simulink model "untitled1"  (Simulink 7.9)
settings: Solver=ode45  StartTime=0.0  StopTime=1  RelTol=1e-3
values from neighbouring files (symbols this model uses):
  D = [  1 -1  1 -1  1  1 -1 -1 ... (first row only)    [cdma.m]    (also in compressed_sampling.m = idct(eye(5000,5000)))
  j = imread('lena.jpg')    [ansk3.m]    (also in cosine_filter.m = 2; imag1.m)
undefined symbols (not defined in the file or in its folder): dfilt, F_nco, OFDM_Frame, Pilot_Level, QAM_Level
libraries: dspobslib x4, dspsigops x4, simulink x2, dsparch4 x1, commrandsrc2 x1, dspxfrm3 x1, commdigbbndam3 x1, dspstat3 x1
settings Model: Creator=ArunKB

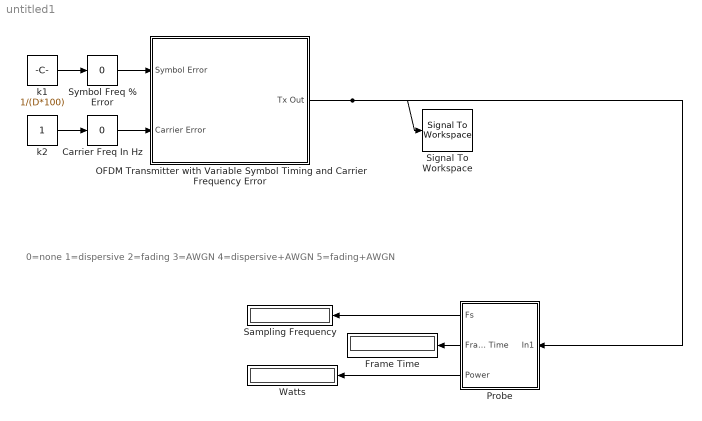
== system untitled1 ==
  note: 0=none
      | 1=dispersive
      | 2=fading
      | 3=AWGN
      | 4=dispersive+AWGN
      | 5=fading+AWGN
  Carrier Freq In Hz : simulink/Math Operations/Slider Gain  low=-1000  gain=0  high=1000
  Frame Time : Display
  OFDM Transmitter with Variable Symbol Timing and Carrier Frequency Error : Subsystem
  Probe : Subsystem
  Sampling Frequency : Display
  Signal To Workspace : SignalToWorkspace  VariableName=yout
      settings: CopyFcn=dspblkcopystw(gcbh);
  "Symbol Freq % Error " : simulink/Math Operations/Slider Gain  low=-0.5  gain=0  high=0.5
  Watts : Display
  k1 : Constant  Value=1/(D*100)
  k2 : Constant
  wires:
  k1/1 -> "Symbol Freq % Error "/1
  "Symbol Freq % Error "/1 -> OFDM Transmitter with Variable Symbol Timing and Carrier Frequency Error/1(Symbol Error)
  k2/1 -> Carrier Freq In Hz/1
  Carrier Freq In Hz/1 -> OFDM Transmitter with Variable Symbol Timing and Carrier Frequency Error/2(Carrier Error)
  OFDM Transmitter with Variable Symbol Timing and Carrier Frequency Error/1(Tx Out) -> Signal To Workspace/1, Probe/1(In1)
  Probe/1(Fs) -> Sampling Frequency/1
  Probe/3(Power) -> Watts/1
  Probe/2(Frame Time) -> Frame Time/1

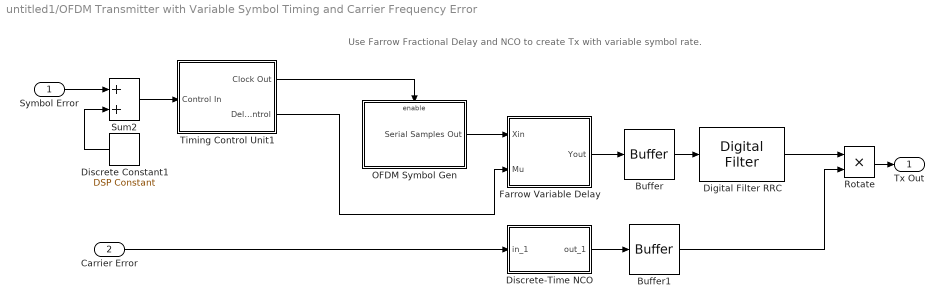
== system untitled1/OFDM Transmitter with Variable Symbol Timing and Carrier Frequency Error ==
  note: Use Farrow Fractional Delay and NCO to create Tx with variable symbol rate.
  Symbol Error : Inport
  Carrier Error : Inport  Port=2
  Buffer : Buffer  N=OFDM_Frame*D
  Buffer1 : Buffer  N=OFDM_Frame*D
  "Digital Filter RRC " : dsparch4/Digital Filter  TypePopup=FIR (all zeros)  IIRFiltStruct=Direct form II transposed  AllPoleFiltStruct=Direct form  FIRFiltStruct=Direct form  CoeffSource=Specify via dialog  NumCoeffs=rrc_coef  DenCoeffs=[1 0.1]  BiQuadCoeffs=[1 0.3 0.4 1 0.1 0.2]  LatticeCoeffs=[0.2 0.4]  denIgnore=on  FiltPerSampPopup=One filter per frame  IC=0  ICnum=0  ICden=0  roundingMode=Floor  overflowMode=off  ScaleValues=1  scaleValueFracLength=14  stageInFracLength=15  stageOutFracLength=15  FilterSource=Specify via dialog  dfiltObjectName=dfilt.dffir([1 2 1])  InputProcessing=Inherited (this choice will be removed - see release notes)
  Discrete Constant1 : dspobslib/DSP Constant  Value=1/D  SampleMode=Discrete  discreteOutput=Sample-based (interpret vectors as 1-D)  continuousOutput=Sample-based  sampTime=inf  framePeriod=inf  dataType=Inherit via back propagation  isSigned=on  wordLen=16  udDataType=sfix(16)  fracBitsMode=Best precision  numFracBits=15  InterpretAs1D=on  Ts=inf  FramebasedOutput=off
      settings: additionalParams=on
  Discrete-Time NCO : Subsystem  mask(Discrete-Time VCO){Ac=1, Fc=0, Kc=1, Ph=0, ts=1/F_nco}
      mask prompts: Ac "Output amplitude:"; Fc "Oscillation frequency (Hz):"; Kc "Input sensitivity:"; Ph "Initial phase (rad):"; ts "Sample time:"
      mask help: Generate a discrete-time output signal whose frequency changes in response to the amplitude variations of the input signal. The input signal must be a scalar.
      mask init:
      | if ((length(Ac)~=1) | (length(Fc)~=1) | (length(Kc)~=1) | (length(Ph)~=1) | (length(ts)~=1) |(length(Ph)~=1))error('Mask parameters must be scalar values.');end;
      | pi2=2*pi;
      mask Help: helpview(commbhelp)
      mask Display: disp('Discrete-Time\nNCO (rab)')
  Farrow Variable Delay : Subsystem
  OFDM Symbol Gen : Subsystem
  Rotate : Product  RndMeth=Zero
  Sum2 : Sum  SaturateOnIntegerOverflow=on  InputSameDT=on  OutDataTypeStr=Inherit: Same as first input
  Timing Control Unit1 : Subsystem
  Tx Out : Outport
  wires:
  Rotate/1 -> Tx Out/1
  Symbol Error/1 -> Sum2/1
  Farrow Variable Delay/1(Yout) -> Buffer/1
  Buffer/1 -> "Digital Filter RRC "/1
  "Digital Filter RRC "/1 -> Rotate/1
  Discrete-Time NCO/1(out_1) -> Buffer1/1
  Carrier Error/1 -> Discrete-Time NCO/1(in_1)
  Buffer1/1 -> Rotate/2
  Sum2/1 -> Timing Control Unit1/1(Control In)
  Timing Control Unit1/2(Delay Control) -> Farrow Variable Delay/2(Mu)
  Timing Control Unit1/1(Clock Out) -> OFDM Symbol Gen/Enable
  Discrete Constant1/1 -> Sum2/2
  OFDM Symbol Gen/1(Serial Samples Out) -> Farrow Variable Delay/1(Xin)

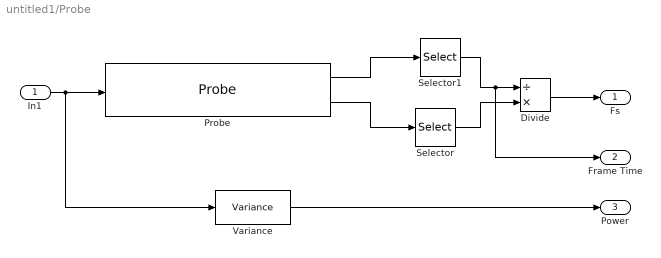
== system untitled1/Probe ==
  In1 : Inport
  Divide : Product  Inputs=/*
  Probe : Probe  ProbeWidth=off  ProbeComplexSignal=off  ProbeSignalDimensions=on
  Selector : Selector  InputPortWidth=2  IndexOptions=Index vector (dialog)  Indices=[1]  OutputSizes=1
  Selector1 : Selector  InputPortWidth=2  IndexOptions=Index vector (dialog)  Indices=[1]  OutputSizes=1
  Variance : dspstat3/Variance  run=off  reset_popup=None  InputProcessing=Columns as channels (frame based)  directionMode=Each column  dimension=1  treatSBRowAsCol=on  roiEnable=off  roiType=Rectangles  roiPortion=Entire ROI  roiOutput=Individual statistics for each ROI  roiFlag=off  roundingMode=Floor  overflowMode=off
  Fs : Outport
  Frame Time : Outport  Port=2
  Power : Outport  Port=3
  wires:
  In1/1 -> Probe/1, Variance/1
  Divide/1 -> Fs/1
  Selector/1 -> Divide/2
  Selector1/1 -> Divide/1, Frame Time/1
  Probe/1 -> Selector1/1
  Probe/2 -> Selector/1
  Variance/1 -> Power/1

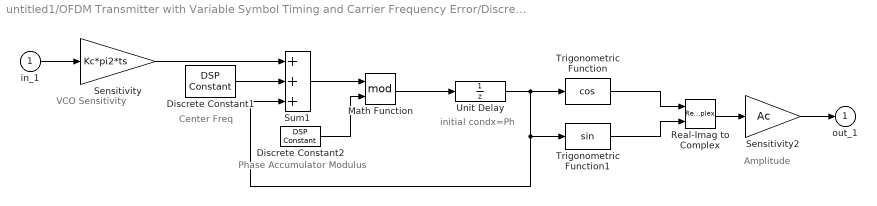
== system untitled1/OFDM Transmitter with Variable Symbol Timing and Carrier Frequency Error/Discrete-Time NCO ==
  note: initial condx=Ph
  note: VCO Sensitivity
  note: Center Freq
  note: Phase Accumulator
      | Modulus
  note: Amplitude
  in_1 : Inport
  Discrete Constant1 : dspobslib/DSP Constant  Value=Fc*pi2*ts  SampleMode=Discrete  discreteOutput=Sample-based (interpret vectors as 1-D)  continuousOutput=Sample-based  sampTime=ts  framePeriod=ts  dataType=Inherit via back propagation  isSigned=on  wordLen=16  udDataType=sfix(16)  fracBitsMode=Best precision  numFracBits=15  InterpretAs1D=on  Ts=ts  FramebasedOutput=off
      settings: additionalParams=on
  Discrete Constant2 : dspobslib/DSP Constant  Value=pi2  SampleMode=Discrete  discreteOutput=Sample-based (interpret vectors as 1-D)  continuousOutput=Sample-based  sampTime=ts  framePeriod=ts  dataType=Inherit via back propagation  isSigned=on  wordLen=16  udDataType=sfix(16)  fracBitsMode=Best precision  numFracBits=15  InterpretAs1D=on  Ts=ts  FramebasedOutput=off
      settings: additionalParams=on
  Math Function : Math  Operator=mod  SaturateOnIntegerOverflow=on
  Real-Imag to Complex : RealImagToComplex
  Sensitivity : Gain  Gain=Kc*pi2*ts  SaturateOnIntegerOverflow=on  OutDataTypeStr=Inherit: Same as input  ParamDataTypeStr=Inherit: Same as input
  Sensitivity2 : Gain  Gain=Ac  SaturateOnIntegerOverflow=on  OutDataTypeStr=Inherit: Same as input  ParamDataTypeStr=Inherit: Same as input
  Sum1 : Sum  Inputs=+++  SaturateOnIntegerOverflow=on  InputSameDT=on  OutDataTypeStr=Inherit: Same as first input
  Trigonometric Function : Trigonometry  Operator=cos
  Trigonometric Function1 : Trigonometry
  Unit Delay : UnitDelay  X0=Ph  SampleTime=ts
  out_1 : Outport  InitialOutput=0
  wires:
  Real-Imag to Complex/1 -> Sensitivity2/1
  Trigonometric Function1/1 -> Real-Imag to Complex/2
  Discrete Constant2/1 -> Math Function/2
  Sum1/1 -> Math Function/1
  Math Function/1 -> Unit Delay/1
  in_1/1 -> Sensitivity/1
  Sensitivity/1 -> Sum1/1
  Unit Delay/1 -> Trigonometric Function/1, Trigonometric Function1/1, Sum1/3
  Trigonometric Function/1 -> Real-Imag to Complex/1
  Sensitivity2/1 -> out_1/1
  Discrete Constant1/1 -> Sum1/2

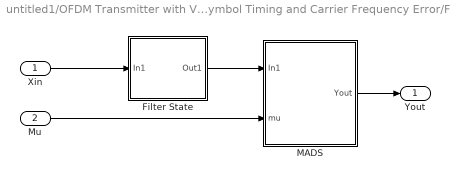
== system untitled1/OFDM Transmitter with Variable Symbol Timing and Carrier Frequency Error/Farrow Variable Delay ==
  Xin : Inport
  Mu : Inport  Port=2
  Filter State : Subsystem
  MADS : Subsystem
  Yout : Outport
  wires:
  Filter State/1(Out1) -> MADS/1(In1)
  Xin/1 -> Filter State/1(In1)
  Mu/1 -> MADS/2(mu)
  MADS/1(Yout) -> Yout/1

== system untitled1/OFDM Transmitter with Variable Symbol Timing and Carrier Frequency Error/OFDM Symbol Gen ==
  note: Output Samples Serially
  note: Note: Ouptut is SET TO ZERO
      | when not enabled.
      | This effecitvly inserts ZEROS in the stream
      | for proper interpolation.
  Enable : EnablePort
  Divide by  OFDM_Frame length : Subsystem  TreatAsAtomicUnit=on  mask(Pulse Divider){div=OFDM_Frame, ph=0}
      mask prompts: div "Modulo:"; ph "Initial Phase Delay (cycles):"
  OFDM Generator : Subsystem
  Selector : Selector  InputPortWidth=80  IndexOptions=Index vector (port)  Indices=[1 3]  OutputSizes=1
  Serial Samples Out : Outport  OutputWhenDisabled=reset  InitialOutput=0+j*eps
  wires:
  OFDM Generator/1(Out1) -> Selector/1
  Divide by  OFDM_Frame length/1(Enable) -> OFDM Generator/Enable
  Selector/1 -> Serial Samples Out/1
  Divide by  OFDM_Frame length/2(Count) -> Selector/2

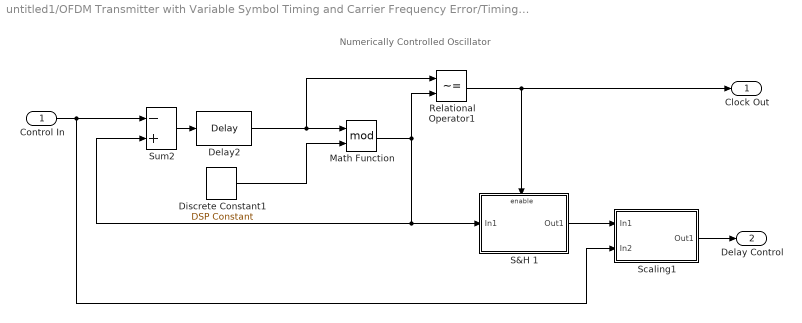
== system untitled1/OFDM Transmitter with Variable Symbol Timing and Carrier Frequency Error/Timing Control Unit1 ==
  note: Numerically Controlled Oscillator
  Control In : Inport
  Delay2 : dspsigops/Delay  InputProcessing=Inherited (this choice will be removed - see release notes)  dly_unit=Samples  delay=1  ic_detail=on  dif_ic_for_ch=off  dif_ic_for_dly=off  ic=0  reset_popup=None
  Discrete Constant1 : dspobslib/DSP Constant  Value=1  SampleMode=Discrete  discreteOutput=Sample-based (interpret vectors as 1-D)  continuousOutput=Sample-based  sampTime=inf  framePeriod=inf  dataType=Inherit via back propagation  isSigned=on  wordLen=16  udDataType=sfix(16)  fracBitsMode=Best precision  numFracBits=15  InterpretAs1D=on  Ts=inf  FramebasedOutput=off
      settings: additionalParams=on
  Math Function : Math  Operator=mod  SaturateOnIntegerOverflow=on
  Relational Operator1 : RelationalOperator  Operator=~=  OutDataTypeStr=boolean
  S&H 1 : Subsystem  TreatAsAtomicUnit=on
  Scaling1 : Subsystem
  Sum2 : Sum  Inputs=-+  SaturateOnIntegerOverflow=on  InputSameDT=on  OutDataTypeStr=Inherit: Same as first input
  Clock Out : Outport
  Delay Control : Outport  Port=2
  wires:
  Scaling1/1(Out1) -> Delay Control/1
  S&H 1/1(Out1) -> Scaling1/1(In1)
  Delay2/1 -> Math Function/1, Relational Operator1/1
  Discrete Constant1/1 -> Math Function/2
  Sum2/1 -> Delay2/1
  Math Function/1 -> Relational Operator1/2, S&H 1/1(In1), Sum2/2
  Relational Operator1/1 -> Clock Out/1, S&H 1/Enable
  Control In/1 -> Sum2/1, Scaling1/2(In2)

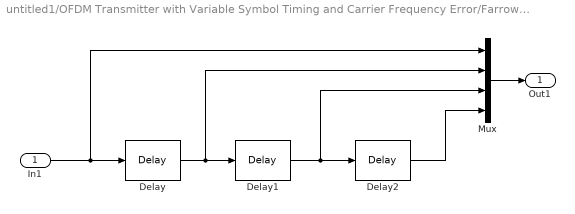
== system untitled1/OFDM Transmitter with Variable Symbol Timing and Carrier Frequency Error/Farrow Variable Delay/Filter State ==
  In1 : Inport
  Delay : dspsigops/Delay  InputProcessing=Inherited (this choice will be removed - see release notes)  dly_unit=Samples  delay=1  ic_detail=off  dif_ic_for_ch=off  dif_ic_for_dly=off  ic=0  reset_popup=None
  Delay1 : dspsigops/Delay  InputProcessing=Inherited (this choice will be removed - see release notes)  dly_unit=Samples  delay=1  ic_detail=off  dif_ic_for_ch=off  dif_ic_for_dly=off  ic=0  reset_popup=None
  Delay2 : dspsigops/Delay  InputProcessing=Inherited (this choice will be removed - see release notes)  dly_unit=Samples  delay=1  ic_detail=off  dif_ic_for_ch=off  dif_ic_for_dly=off  ic=0  reset_popup=None
  Mux : Mux
  Out1 : Outport
  wires:
  In1/1 -> Delay/1, Mux/1
  Delay/1 -> Mux/2, Delay1/1
  Delay1/1 -> Mux/3, Delay2/1
  Delay2/1 -> Mux/4
  Mux/1 -> Out1/1

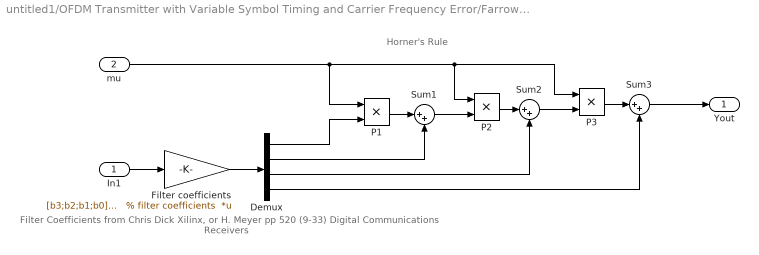
== system untitled1/OFDM Transmitter with Variable Symbol Timing and Carrier Frequency Error/Farrow Variable Delay/MADS ==
  note: Horner's Rule
  note: Filter Coefficients from Chris Dick Xilinx,
      | or H. Meyer pp 520 (9-33) Digital Communications Receivers
  In1 : Inport
  mu : Inport  Port=2
  Demux : Demux
  Filter coefficients : Gain  Gain="[b3;b2;b1;b0]   % filter coefficients"  Multiplication=Matrix(K*u)  SaturateOnIntegerOverflow=on  OutDataTypeStr=Inherit: Same as input  ParamDataTypeStr=Inherit: Same as input
  P1 : Product  SaturateOnIntegerOverflow=on  OutDataTypeStr=Inherit: Same as first input
  P2 : Product  SaturateOnIntegerOverflow=on  OutDataTypeStr=Inherit: Same as first input
  P3 : Product  SaturateOnIntegerOverflow=on  OutDataTypeStr=Inherit: Same as first input
  Sum1 : Sum  Inputs=|++  SaturateOnIntegerOverflow=on
  Sum2 : Sum  Inputs=|++  SaturateOnIntegerOverflow=on
  Sum3 : Sum  Inputs=|++  SaturateOnIntegerOverflow=on
  Yout : Outport
  wires:
  P3/1 -> Sum3/1
  P2/1 -> Sum2/1
  Filter coefficients/1 -> Demux/1
  In1/1 -> Filter coefficients/1
  mu/1 -> P3/1, P2/1, P1/1
  Demux/1 -> P1/2
  Sum1/1 -> P2/2
  Sum2/1 -> P3/2
  Demux/2 -> Sum1/2
  P1/1 -> Sum1/1
  Demux/3 -> Sum2/2
  Demux/4 -> Sum3/2
  Sum3/1 -> Yout/1

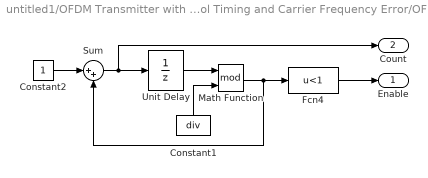
== system untitled1/OFDM Transmitter with Variable Symbol Timing and Carrier Frequency Error/OFDM Symbol Gen/Divide by  OFDM_Frame length ==
  Constant1 : Constant  Value=div
  Constant2 : Constant
  Fcn4 : Fcn  Expr=u<1
  Math Function : Math  Operator=mod  SaturateOnIntegerOverflow=on
  Sum : Sum  Inputs=|++  SaturateOnIntegerOverflow=on  InputSameDT=on  OutDataTypeStr=Inherit: Same as first input
  Unit Delay : UnitDelay  X0=div-ph  SampleTime=-1
  Enable : Outport
  Count : Outport  Port=2
  wires:
  Sum/1 -> Unit Delay/1, Count/1
  Constant2/1 -> Sum/1
  Unit Delay/1 -> Math Function/1
  Math Function/1 -> Sum/2, Fcn4/1
  Constant1/1 -> Math Function/2
  Fcn4/1 -> Enable/1

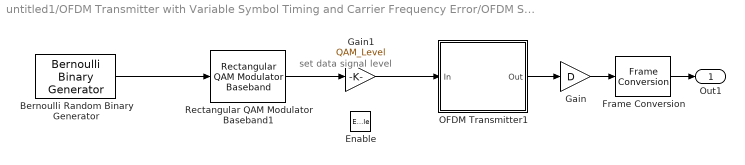
== system untitled1/OFDM Transmitter with Variable Symbol Timing and Carrier Frequency Error/OFDM Symbol Gen/OFDM Generator ==
  note: set data signal level
  Enable : EnablePort
  Bernoulli Random Binary Generator : commrandsrc2/Bernoulli Binary Generator  P=0.5  seed=123  Ts=-1  frameBased=on  sampPerFrame=Bits_per_Frame  orient=off  outDataType=double
  Frame Conversion : FrameConversion  OutFrame=Sample-based
  Gain : Gain  Gain=D
  Gain1 : Gain  Gain=QAM_Level  SaturateOnIntegerOverflow=on  OutDataTypeStr=Inherit: Same as input  ParamDataTypeStr=Inherit: Same as input
  OFDM Transmitter1 : Subsystem
      mask Display: disp('OFDM\nTransmitter')
  Rectangular QAM Modulator Baseband1 : commdigbbndam3/Rectangular QAM Modulator Baseband  M=4  InType=Bit  Enc=Binary  Mapping=[0:15]  PowType=Min. distance between symbols  MinDist=2  AvgPow=1  PeakPow=1  Ph=0  outDtype=double  outWordLen=16  outUDDataType=sfix(16)  outFracLenMode=Best precision  outFracLen=15
  Out1 : Outport
  wires:
  Bernoulli Random Binary Generator/1 -> Rectangular QAM Modulator Baseband1/1
  OFDM Transmitter1/1(Out) -> Gain/1
  Rectangular QAM Modulator Baseband1/1 -> Gain1/1
  Gain/1 -> Frame Conversion/1
  Gain1/1 -> OFDM Transmitter1/1(In)
  Frame Conversion/1 -> Out1/1

== system untitled1/OFDM Transmitter with Variable Symbol Timing and Carrier Frequency Error/Timing Control Unit1/S&H 1 ==
  In1 : Inport
  Enable : EnablePort
  Out1 : Outport
  wires:
  In1/1 -> Out1/1

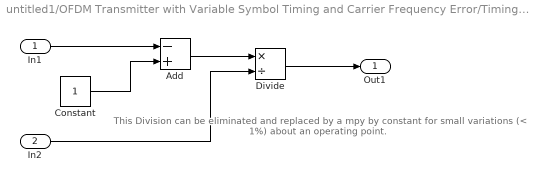
== system untitled1/OFDM Transmitter with Variable Symbol Timing and Carrier Frequency Error/Timing Control Unit1/Scaling1 ==
  note: This Division can be eliminated
      | and replaced by a mpy by constant
      | for small variations (< 1%)
      | about an operating point.
  In1 : Inport
  In2 : Inport  Port=2
  Add : Sum  Inputs=-+
  Constant : Constant
  Divide : Product  Inputs=*/
  Out1 : Outport
  wires:
  In2/1 -> Divide/2
  In1/1 -> Add/1
  Constant/1 -> Add/2
  Add/1 -> Divide/1
  Divide/1 -> Out1/1

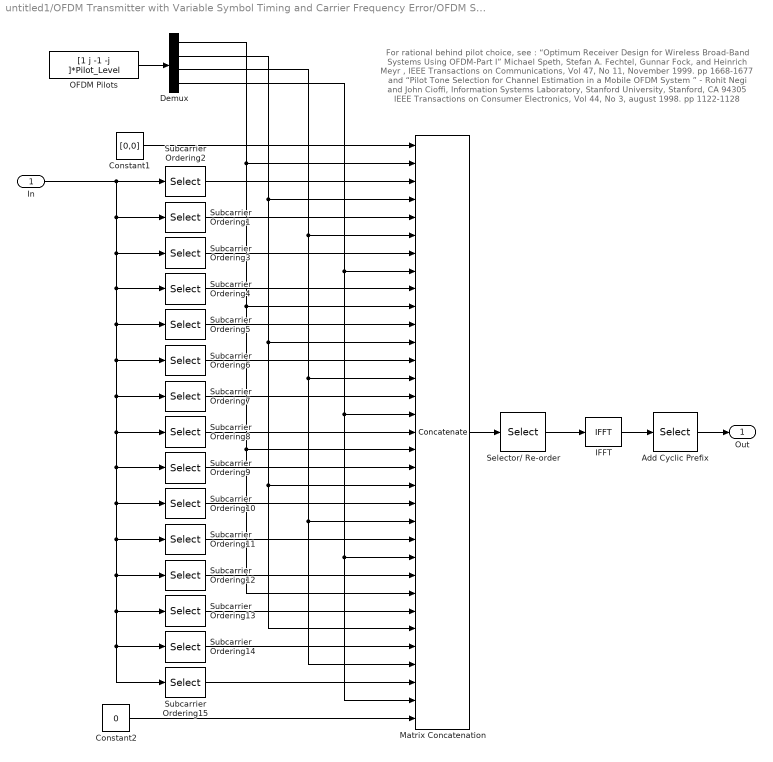
== system untitled1/OFDM Transmitter with Variable Symbol Timing and Carrier Frequency Error/OFDM Symbol Gen/OFDM Generator/OFDM Transmitter1 ==
  note: For rational behind pilot choice, see :
      | “Optimum Receiver Design for Wireless Broad-Band Systems Using OFDM-Part I”
      | Michael Speth, Stefan A. Fechtel, Gunnar Fock, and Heinrich Meyr ,
      |  IEEE Transactions on Communications, Vol 47, No 11, November 1999. pp 1668-1677
      | and
      | “Pilot Tone Selection for Channel Estimation in a Mobile OFDM System ” -
      |  Rohit Negi and John Cioffi, Information Systems Laboratory, Stanford University, Stanford, CA 94305
      | IEEE Transactions on Consumer Electronics, Vol 44, No 3, august 1998. pp 1122-1128
  In : Inport
  Add Cyclic Prefix : Selector  InputPortWidth=64  IndexOptions=Index vector (dialog)  Indices=[49:64 1:64]  OutputSizes=1
  Constant1 : Constant  Value=[0,0]
  Constant2 : Constant  Value=0
  Demux : Demux
  IFFT : dspxfrm3/IFFT  CompMethod=Table lookup  TableOpt=HYBRID  TableOptActive=Speed  BitRevOrder=off  cs_in=off  SkipNorm=on  InheritFFTLength=on  FFTLength=64  mode=Complex  outSamplingMode=Frame based  RowConvenienceOn=on  FFTImplementation=Auto  firstCoeffDataTypeStr=Inherit: Same word length as input  firstCoeffLastDataTypeStr=Inherit: Same word length as input  outputMin=[]  outputMax=[]  roundingMode=Floor  overflowMode=off
  Matrix Concatenation : Concatenate  NumInputs=33  Mode=Multidimensional array
  OFDM Pilots : Constant  Value="[1 j -1 -j   ]*Pilot_Level"
  Selector/ Re-order : Selector  InputPortWidth=64  IndexOptions=Index vector (dialog)  Indices=[33:64 1:32]  OutputSizes=1
  Subcarrier Ordering1 : Selector  InputPortWidth=Symbols_per_Frame  IndexOptions=Index vector (dialog)  Indices=4:6  OutputSizes=1
  Subcarrier Ordering10 : Selector  InputPortWidth=Symbols_per_Frame  IndexOptions=Index vector (dialog)  Indices=28:30  OutputSizes=1
  Subcarrier Ordering11 : Selector  InputPortWidth=Symbols_per_Frame  IndexOptions=Index vector (dialog)  Indices=31:33  OutputSizes=1
  Subcarrier Ordering12 : Selector  InputPortWidth=Symbols_per_Frame  IndexOptions=Index vector (dialog)  Indices=34:36  OutputSizes=1
  Subcarrier Ordering13 : Selector  InputPortWidth=Symbols_per_Frame  IndexOptions=Index vector (dialog)  Indices=37:39  OutputSizes=1
  Subcarrier Ordering14 : Selector  InputPortWidth=Symbols_per_Frame  IndexOptions=Index vector (dialog)  Indices=40:42  OutputSizes=1
  Subcarrier Ordering15 : Selector  InputPortWidth=Symbols_per_Frame  IndexOptions=Index vector (dialog)  Indices=43:45  OutputSizes=1
  Subcarrier Ordering2 : Selector  InputPortWidth=Symbols_per_Frame  IndexOptions=Index vector (dialog)  Indices=1:3  OutputSizes=1
  Subcarrier Ordering3 : Selector  InputPortWidth=Symbols_per_Frame  IndexOptions=Index vector (dialog)  Indices=7:9  OutputSizes=1
  Subcarrier Ordering4 : Selector  InputPortWidth=Symbols_per_Frame  IndexOptions=Index vector (dialog)  Indices=10:12  OutputSizes=1
  Subcarrier Ordering5 : Selector  InputPortWidth=Symbols_per_Frame  IndexOptions=Index vector (dialog)  Indices=13:15  OutputSizes=1
  Subcarrier Ordering6 : Selector  InputPortWidth=Symbols_per_Frame  IndexOptions=Index vector (dialog)  Indices=16:18  OutputSizes=1
  Subcarrier Ordering7 : Selector  InputPortWidth=Symbols_per_Frame  IndexOptions=Index vector (dialog)  Indices=19:21  OutputSizes=1
  Subcarrier Ordering8 : Selector  InputPortWidth=Symbols_per_Frame  IndexOptions=Index vector (dialog)  Indices=22:24  OutputSizes=1
  Subcarrier Ordering9 : Selector  InputPortWidth=Symbols_per_Frame  IndexOptions=Index vector (dialog)  Indices=25:27  OutputSizes=1
  Out : Outport
  wires:
  In/1 -> Subcarrier Ordering14/1, Subcarrier Ordering15/1, Subcarrier Ordering13/1, Subcarrier Ordering12/1, Subcarrier Ordering11/1, Subcarrier Ordering10/1, Subcarrier Ordering9/1, Subcarrier Ordering8/1, Subcarrier Ordering7/1, Subcarrier Ordering6/1, Subcarrier Ordering5/1, Subcarrier Ordering4/1, Subcarrier Ordering3/1, Subcarrier Ordering1/1, Subcarrier Ordering2/1
  IFFT/1 -> Add Cyclic Prefix/1
  Matrix Concatenation/1 -> Selector/ Re-order/1
  Selector/ Re-order/1 -> IFFT/1
  Subcarrier Ordering2/1 -> Matrix Concatenation/3
  Subcarrier Ordering1/1 -> Matrix Concatenation/5
  Subcarrier Ordering3/1 -> Matrix Concatenation/7
  Subcarrier Ordering4/1 -> Matrix Concatenation/9
  Subcarrier Ordering5/1 -> Matrix Concatenation/11
  Subcarrier Ordering6/1 -> Matrix Concatenation/13
  Subcarrier Ordering7/1 -> Matrix Concatenation/15
  Subcarrier Ordering8/1 -> Matrix Concatenation/17
  Subcarrier Ordering9/1 -> Matrix Concatenation/19
  Subcarrier Ordering10/1 -> Matrix Concatenation/21
  Subcarrier Ordering11/1 -> Matrix Concatenation/23
  Subcarrier Ordering12/1 -> Matrix Concatenation/25
  Subcarrier Ordering13/1 -> Matrix Concatenation/27
  Subcarrier Ordering14/1 -> Matrix Concatenation/29
  Subcarrier Ordering15/1 -> Matrix Concatenation/31
  Add Cyclic Prefix/1 -> Out/1
  Constant1/1 -> Matrix Concatenation/1
  Constant2/1 -> Matrix Concatenation/33
  Demux/2 -> Matrix Concatenation/4, Matrix Concatenation/12, Matrix Concatenation/20, Matrix Concatenation/28
  Demux/3 -> Matrix Concatenation/6, Matrix Concatenation/14, Matrix Concatenation/22, Matrix Concatenation/30
  Demux/4 -> Matrix Concatenation/8, Matrix Concatenation/16, Matrix Concatenation/24, Matrix Concatenation/32
  OFDM Pilots/1 -> Demux/1
  Demux/1 -> Matrix Concatenation/26, Matrix Concatenation/18, Matrix Concatenation/10, Matrix Concatenation/2
